simulink model "NetworkingModel"  (R2024a)
settings: Solver=VariableStepAuto  StartTime=0.0  StopTime=10.0  RelTol=1e-3
libraries: commchan3 x2
settings Model: Creator=sampa  LastModifiedBy=sampa

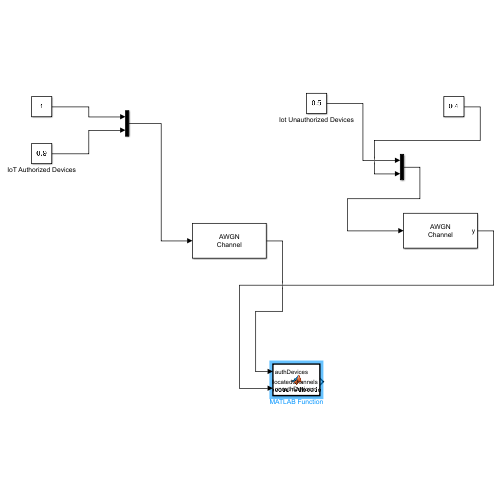
[thumbnail: Simulink's stored preview of the top-level diagram]
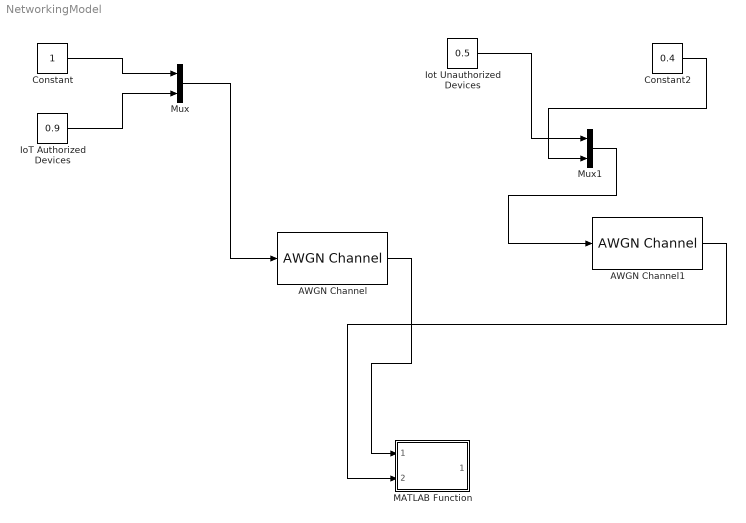
== system NetworkingModel ==
  AWGN Channel : commchan3/AWGN Channel  LegacyMode=off  NoiseMethod="Signal to noise ratio  (SNR)"  noiseMode="Signal to noise ratio  (SNR)"  EbNo=10  EsNo=10  SNR=20  BitsPerSymbol=1  SignalPower=1  SamplesPerSymbol=1  SymbolPeriod=1  VarianceSource=Parameter  Variance=1  RandomStream=Global stream  Seed=67  SimulateUsing=Code generation
  AWGN Channel1 : commchan3/AWGN Channel  LegacyMode=off  NoiseMethod="Signal to noise ratio  (SNR)"  noiseMode="Signal to noise ratio  (SNR)"  EbNo=10  EsNo=10  SNR=10  BitsPerSymbol=1  SignalPower=1  SamplesPerSymbol=1  SymbolPeriod=1  VarianceSource=Parameter  Variance=1  RandomStream=Global stream  Seed=67  SimulateUsing=Code generation
  Constant : Constant
  Constant2 : Constant  Value=0.4
  IoT Authorized Devices : Constant  Value=0.9
  Iot Unauthorized Devices : Constant  Value=0.5
  MATLAB Function : MATLAB Function  TreatAsAtomicUnit=on
  Mux : Mux  Inputs=2
  Mux1 : Mux  Inputs=2
  wires:
  IoT Authorized Devices/1 -> Mux/2
  Constant/1 -> Mux/1
  Mux/1 -> AWGN Channel/1
  Iot Unauthorized Devices/1 -> Mux1/1
  Constant2/1 -> Mux1/2
  Mux1/1 -> AWGN Channel1/1
  AWGN Channel/1 -> MATLAB Function/1(authDevices)
  AWGN Channel1/1 -> MATLAB Function/2(unauthDevices)

== matlab function NetworkingModel/MATLAB Function ==
  data: authDevices input; allocatedChannels output; unauthDevices input
function allocatedChannels = spectrumAllocation(authDevices, unauthDevices)
    % Inputs: authDevices, unauthDevices
    % authDevices: Signals from authorized IoT devices
    % unauthDevices: Signals from unauthorized IoT devices

    % Example Allocation Logic
    allocatedChannels = zeros(4, 1); % Initialize output for 6 devices

    % Prioritize authorized devices
    for i = 1:2 % First three are authorized devices
        if authDevices(i) > 0.7 % Threshold for active devices
            allocatedChannels(i) = 1; % Allocate channel
        end
    end

    % Allocate remaining channels to unauthorized devices
    for j = 3:4 % Next three are unauthorized devices
        if unauthDevices(j-2) > 0.3 % Lower threshold for unauthorized
            allocatedChannels(j) = 1; % Allocate channel
        end
    end
end
